simulink model "DiagramaBloquesSistMecanico"  (R2023b)
settings: Solver=VariableStepAuto  StartTime=0.0  StopTime=10.0  RelTol=1e-3
values from neighbouring files (symbols this model uses):
  b_eq = b_m + b_l/(r^2)    (= 2.19444444444e-05)    [Parametros.m]
  g = 9.80665    [Parametros.m]
  J_eq = J_m + J_l/(r^2)    [Parametros.m]
  k_l = m*l_cm + m_l(1)*l_l    [Parametros.m]
  r = 120    [Parametros.m]
settings Model: Creator=Home  LastModifiedBy=Home

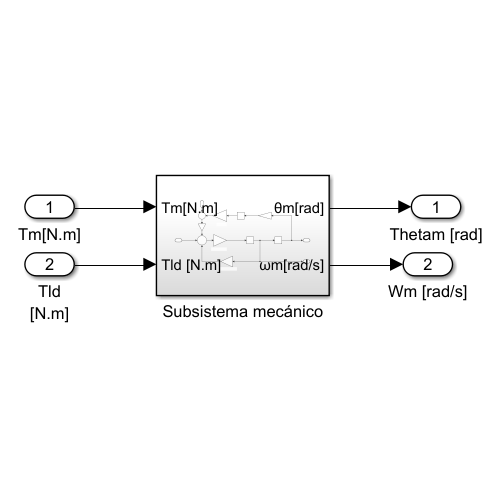
[thumbnail: Simulink's stored preview of the top-level diagram]
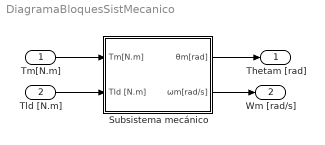
== system DiagramaBloquesSistMecanico ==
  Tm[N.m] : Inport
  Tld [N.m] : Inport  Port=2
  Subsistema mecánico : Subsystem
  Thetam [rad] : Outport
  Wm [rad/s] : Outport  Port=2
  wires:
  Tm[N.m]/1 -> Subsistema mecánico/1(Tm[N.m])
  Tld [N.m]/1 -> Subsistema mecánico/2(Tld [N.m])
  Subsistema mecánico/1(θm[rad]) -> Thetam [rad]/1
  Subsistema mecánico/2(ωm[rad/s]) -> Wm [rad/s]/1

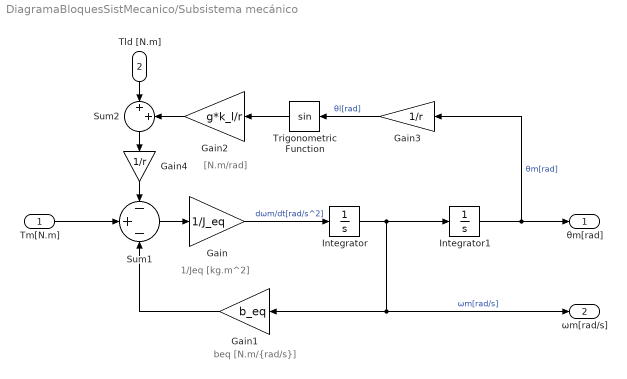
== system DiagramaBloquesSistMecanico/Subsistema mecánico ==
  note: beq [N.m/{rad/s}]
  note: 1/Jeq [kg.m^2]
  note: [N.m/rad]
  Tm[N.m] : Inport
  Tld [N.m] : Inport  Port=2
  Gain : Gain  Gain=1/J_eq
  Gain1 : Gain  Gain=b_eq
  Gain2 : Gain  Gain=g*k_l/r
  Gain3 : Gain  Gain=1/r
  Gain4 : Gain  Gain=1/r
  Integrator : Integrator
  Integrator1 : Integrator
  Sum1 : Sum  Inputs=-+-
  Sum2 : Sum  Inputs=|++
  Trigonometric Function : Trigonometry
  θm[rad] : Outport
  ωm[rad/s] : Outport  Port=2
  wires:
  Gain3/1 -> Trigonometric Function/1  "θl[rad]"
  Tm[N.m]/1 -> Sum1/2
  Integrator/1 -> ωm[rad/s]/1, Gain1/1, Integrator1/1  "ωm[rad/s]"
  Gain4/1 -> Sum1/1
  Integrator1/1 -> θm[rad]/1, Gain3/1  "θm[rad]"
  Trigonometric Function/1 -> Gain2/1
  Gain1/1 -> Sum1/3
  Gain/1 -> Integrator/1  "dωm/dt[rad/s^2]"
  Sum1/1 -> Gain/1
  Tld [N.m]/1 -> Sum2/1
  Sum2/1 -> Gain4/1
  Gain2/1 -> Sum2/2
